simulink model "car_model_5_28_2023"  (R2022b)
settings: Solver=VariableStepAuto  StartTime=0.0  StopTime=15  RelTol=1e-3
values from neighbouring files (symbols this model uses):
  dZ = 0.295    [Startup.m]
  F0z = [0 0]    [Startup.m]
  phi = 45    [Startup.m]
  X = Reference_Signals.Chassis_Position.X.Data(:)    [Simulation_Data_Parse.m]    (also in Vehicle_Sim_Parse.m = Chassis_Signals.InertFrm.Cg.Disp.X.Data(:))
  Y = Reference_Signals.Chassis_Position.Y.Data(:)    [Simulation_Data_Parse.m]    (also in Vehicle_Sim_Parse.m = Chassis_Signals.InertFrm.Cg.Disp.Y.Data(:))
undefined symbols (not defined in the file or in its folder): chassis, DiscIntNeverNeededParam, driver, IMU_accel, IMU_gyro, IMU_mag, powertrain, psi, sensor, sim, sus, suspension, theta, trn, tvs, veh, VEH, whl, Xdot, Ydot, Z, Zdot
libraries: fl_lib x53, nesl_utility x15, vehdynlibtire x10, vehdynlibsuspension x8, EngineCoolingComponents_lib x5, autolibutils x5, sharedtransform x5, dspstat3 x2, simulink x2, slpidlib x2, shared6dof x2, sensorgpslib x1
(part 2 of 9)

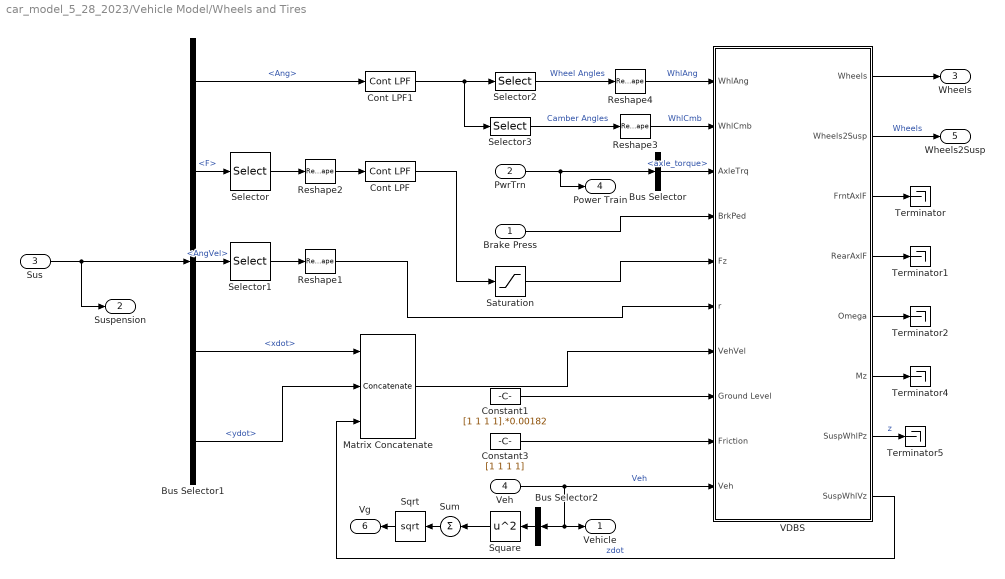
== system car_model_5_28_2023/Vehicle Model/Wheels and Tires ==
  Brake Press : Inport  Unit=Pa
  PwrTrn : Inport  Port=2
  Sus : Inport  Port=3
  Veh : Inport  Port=4
  Bus Selector : BusSelector  OutputSignals=axle_torque
  Bus Selector1 : BusSelector  OutputSignals=Whl.Ang,Whl.F,Whl.AngVel,Whl.xdot,Whl.ydot
  Bus Selector2 : BusSelector  OutputSignals=BdyFrm.Cg.Vel.xdot,BdyFrm.Cg.Vel.ydot  OutputAsBus=on
  Constant1 : Constant  Value=[1 1 1 1].*0.00182
  Constant3 : Constant  Value=[1 1 1 1]
  Cont LPF : autolibutils/Cont LPF  wc=100*2*pi  AbsoluteTolerance=auto  aMode=2
  Cont LPF1 : autolibutils/Cont LPF  wc=100*2*pi  AbsoluteTolerance=auto  aMode=2
  Matrix Concatenate : Concatenate  NumInputs=3  Mode=Multidimensional array
  Reshape{1..4} (4 alike) : Reshape
  Saturation : Saturate  UpperLimit=inf  LowerLimit=-10*9.81*2000  ZeroCross=off
  Selector : Selector  NumberOfDimensions=2  InputPortWidth=3  IndexOptions=Index vector (dialog),Select all  Indices=[3],1  OutputSizes=1,1
  Selector1 : Selector  NumberOfDimensions=2  InputPortWidth=1  IndexOptions=Index vector (dialog),Select all  Indices=[3],1  OutputSizes=1,1
  Selector2 : Selector  NumberOfDimensions=2  InputPortWidth=3  IndexOptions=Index vector (dialog),Select all  Indices=3,1  OutputSizes=1,1
  Selector3 : Selector  NumberOfDimensions=2  InputPortWidth=3  IndexOptions=Index vector (dialog),Select all  Indices=1,1  OutputSizes=1,1
  Sqrt : Sqrt
  Square : Math  Operator=square
  Sum : Sum  Inputs=+
  Terminator{,1..2,4..5} (5 alike) : Terminator
  VDBS : Subsystem  VariantControl=0
  Vehicle : Outport  VectorParamsAs1DForOutWhenUnconnected=off
  Suspension : Outport  Port=2  VectorParamsAs1DForOutWhenUnconnected=off
  Wheels : Outport  Port=3  VectorParamsAs1DForOutWhenUnconnected=off
  Power Train : Outport  Port=4  VectorParamsAs1DForOutWhenUnconnected=off
  Wheels2Susp : Outport  Port=5  VectorParamsAs1DForOutWhenUnconnected=off
  Vg : Outport  Port=6  VectorParamsAs1DForOutWhenUnconnected=off
  wires:
  Bus Selector1/2 -> Selector/1  "<F>"
  VDBS/3(FrntAxlF) -> Terminator/1
  VDBS/4(RearAxlF) -> Terminator1/1
  VDBS/6(Mz) -> Terminator4/1
  Selector1/1 -> Reshape1/1
  Matrix Concatenate/1 -> VDBS/7(VehVel)
  PwrTrn/1 -> Power Train/1, Bus Selector/1
  Reshape4/1 -> VDBS/1(WhlAng)  "WhlAng"
  Reshape3/1 -> VDBS/2(WhlCmb)  "WhlCmb"
  Selector/1 -> Reshape2/1
  Saturation/1 -> VDBS/5(Fz)
  Constant1/1 -> VDBS/8(Ground Level)
  VDBS/8(SuspWhlVz) -> Matrix Concatenate/3  "zdot"
  Bus Selector1/1 -> Cont LPF1/1  "<Ang>"
  Selector3/1 -> Reshape3/1  "Camber Angles"
  Sus/1 -> Suspension/1, Bus Selector1/1
  Bus Selector1/4 -> Matrix Concatenate/1  "<xdot>"
  Bus Selector1/5 -> Matrix Concatenate/2  "<ydot>"
  VDBS/7(SuspWhlPz) -> Terminator5/1  "z"
  Reshape2/1 -> Cont LPF/1
  Bus Selector1/3 -> Selector1/1  "<AngVel>"
  Reshape1/1 -> VDBS/6(r)
  Brake Press/1 -> VDBS/4(BrkPed)
  Constant3/1 -> VDBS/9(Friction)
  Cont LPF/1 -> Saturation/1
  Cont LPF1/1 -> Selector3/1, Selector2/1
  Selector2/1 -> Reshape4/1  "Wheel Angles"
  Veh/1 -> Vehicle/1, Bus Selector2/1, VDBS/10(Veh)  "Veh"
  VDBS/2(Wheels2Susp) -> Wheels2Susp/1  "Wheels"
  VDBS/1(Wheels) -> Wheels/1
  Bus Selector/1 -> VDBS/3(AxleTrq)  "<axle_torque>"
  VDBS/5(Omega) -> Terminator2/1
  Bus Selector2/1 -> Square/1
  Square/1 -> Sum/1
  Sum/1 -> Sqrt/1
  Sqrt/1 -> Vg/1

== system car_model_5_28_2023/Control Systems/TVS/Current Limiting ==
  omega : Inport
  k_TV : Inport  Port=2
  2-D Lookup Table : Lookup_n-D  LookupTableObject=''  BreakpointsForDimension1=tvs.torque_control.omega_bp  BreakpointsForDimension2=tvs.torque_control.k_linear_bp  BreakpointsForDimension1FirstPoint=10  BreakpointsForDimension2FirstPoint=10  BreakpointsForDimension1Spacing=12  BreakpointsForDimension2Spacing=12  Table=tvs.torque_control.k_actual  ExtrapMethod=Clip  DiagnosticForOutOfRangeInput=Error  InternalRulePriority=Speed  RndMeth=Simplest
      settings: InputPortMap=u0,u1
  Gain1 : Gain  Gain=powertrain.gearbox.gr
  K_Actual : Outport
  wires:
  2-D Lookup Table/1 -> K_Actual/1
  k_TV/1 -> 2-D Lookup Table/2
  omega/1 -> Gain1/1
  Gain1/1 -> 2-D Lookup Table/1

== system car_model_5_28_2023/Control Systems/TVS/Optimization ==
  note: reduce this limit?
  driver_input : Inport  OutDataTypeStr=double
  obj_gain : Inport  Port=2
  b : Inport  Port=3  OutDataTypeStr=double
  ub : Inport  Port=4  OutDataTypeStr=double
  lb : Inport  Port=5  OutDataTypeStr=double
  Aeq : Inport  Port=6  OutDataTypeStr=double
  beq : Inport  Port=7  OutDataTypeStr=double
  A Dot : DotProduct  OutDataTypeStr=double
  Aeq Dot : DotProduct  OutDataTypeStr=double
  C Caller : CCaller  FunctionName=bigM_func
  Constant : Constant  Value=sim.top_parameters.TVS_ENABLE
  Constant1 : Constant  Value=[1 1 1 1]
  Demux{,1..4} (5 alike) : Demux
  Switch : Switch  Criteria=u2 > Threshold  SaturateOnIntegerOverflow=off  InputSameDT=off
  Tx_RAW_demux : Mux
  Tx_choose : Switch  Criteria=u2 > Threshold  Threshold=2  OutDataTypeStr=double  SaturateOnIntegerOverflow=off  InputSameDT=off
  Tx_deadband : DeadZone  LowerValue=-10*tvs.power_control.dTx  UpperValue=10*tvs.power_control.dTx
  Tx_equal_gain : Gain  Gain=tvs.power_control.ABS_MAX_TORQUE.*sim.top_parameters.MOTOR_ENABLE  OutDataTypeStr=double
  Tx_equal_offset : Bias  Bias=tvs.power_control.ABS_MAX_TORQUE  SaturateOnIntegerOverflow=off
  Tx_initial : Constant  Value=0  OutDataTypeStr=double
  Tx_reverse_offset : Bias  Bias=-tvs.power_control.ABS_MAX_TORQUE  SaturateOnIntegerOverflow=off
  b Add : Sum  OutDataTypeStr=double
  beq Add : Sum  OutDataTypeStr=double
  lb_offset : Bias  Bias=tvs.power_control.ABS_MAX_TORQUE  SaturateOnIntegerOverflow=off
  optimization_offset_A : Constant  Value=tvs.power_control.ABS_MAX_TORQUE  OutDataTypeStr=double
  optimization_offset_Aeq : Constant  Value=tvs.power_control.ABS_MAX_TORQUE  OutDataTypeStr=double
  ub_offset : Bias  Bias=tvs.power_control.ABS_MAX_TORQUE  SaturateOnIntegerOverflow=off
  yaw_error_limit : Constant  Value=tvs.yaw_control.dy  OutDataTypeStr=double
  Tx : Outport
  exitflag : Outport  Port=2
  wires:
  C Caller/1 -> Tx_choose/2, exitflag/1  "exitflag"
  lb/1 -> lb_offset/1  "lb"
  ub/1 -> ub_offset/1  "ub"
  C Caller/2 -> Tx_RAW_demux/1  "TFL"
  C Caller/5 -> Tx_RAW_demux/4  "TRR"
  C Caller/4 -> Tx_RAW_demux/3  "TRL"
  C Caller/3 -> Tx_RAW_demux/2  "TFR"
  Demux/1 -> C Caller/1  "obj_FL"
  Demux/2 -> C Caller/2  "obj_FR"
  Demux/3 -> C Caller/3  "obj_RL"
  Demux/4 -> C Caller/4  "obj_RR"
  Tx_initial/1 -> C Caller/23, C Caller/24, C Caller/25, C Caller/26  "Tx_initial"
  Demux1/1 -> C Caller/19  "ub_FL"
  Demux1/2 -> C Caller/20  "ub_FR"
  Demux1/3 -> C Caller/21  "ub_RL"
  Demux1/4 -> C Caller/22  "ub_RR"
  Demux2/1 -> C Caller/15  "lb_FL"
  Demux2/2 -> C Caller/16  "lb_FR"
  Demux2/3 -> C Caller/17  "lb_RL"
  Demux2/4 -> C Caller/18  "lb_RR"
  Demux3/3 -> C Caller/13  "Aeq_RL"
  Demux3/2 -> C Caller/12  "Aeq_FR"
  Demux3/1 -> C Caller/11  "Aeq_FL"
  Demux3/4 -> C Caller/14  "Aeq_RR"
  Demux4/1 -> C Caller/6  "A_FL"
  Demux4/2 -> C Caller/7  "A_FR"
  Demux4/3 -> C Caller/8  "A_RL"
  Demux4/4 -> C Caller/9  "A_RR"
  ub_offset/1 -> Demux1/1  "ub_b"
  optimization_offset_Aeq/1 -> Aeq Dot/1  "offset"
  optimization_offset_A/1 -> A Dot/1  "offset"
  beq/1 -> beq Add/1  "beq"
  Aeq Dot/1 -> beq Add/2  "Aeq_b"
  b/1 -> b Add/1  "b"
  A Dot/1 -> b Add/2
  yaw_error_limit/1 -> C Caller/27  "yaw_error_limit"
  Tx_RAW_demux/1 -> Tx_choose/1  "Tx_RAW_TV"
  Constant1/1 -> Demux4/1, A Dot/2  "A"
  b Add/1 -> C Caller/5  "b_b"
  obj_gain/1 -> Demux/1  "obj_gain"
  lb_offset/1 -> Demux2/1  "lb_b"
  Aeq/1 -> Demux3/1, Aeq Dot/2  "Aeq"
  beq Add/1 -> C Caller/10  "beq_b"
  Tx_deadband/1 -> Tx/1  "Tx"
  Tx_reverse_offset/1 -> Tx_deadband/1
  driver_input/1 -> Tx_equal_gain/1
  Tx_choose/1 -> Switch/1
  Tx_equal_gain/1 -> Tx_equal_offset/1  "Tx_equal"
  Tx_equal_offset/1 -> Switch/3, Tx_choose/3
  Switch/1 -> Tx_reverse_offset/1
  Constant/1 -> Switch/2

== system car_model_5_28_2023/Control Systems/TVS/Power Controller ==
  note: Max Throttle as Limit or Max Current as limit?
  note: Tune the endpoints
  vel : Inport  OutDataTypeStr=double
  battery_voltage : Inport  Port=2
  dcl : Inport  Port=3  OutDataTypeStr=double  LockScale=on
  ccl : Inport  Port=4  OutDataTypeStr=double  LockScale=on
  driver_input : Inport  Port=5  OutDataTypeStr=double  LockScale=on
  motor_temp : Inport  Port=6
  mc_temp : Inport  Port=7
  omega : Inport  Port=8
  In9 : Inport  Port=9
  Constant2 : Constant  Value=tvs.power_control.ABS_MIN_TORQUE  OutDataTypeStr=double
  Constant3 : Constant  Value=tvs.power_control.ABS_MAX_TORQUE
  Current to RAW Throttle : Gain  Gain=tvs.power_control.ABS_MAX_TRQ_CMD/tvs.power_control.ABS_MAX_I_FLOW
  Gain : Gain  Gain=tvs.power_control.ABS_MAX_I_FLOW
  Gain4 : Gain  Gain=-sim.top_parameters.MOTOR_ENABLE  ParamDataTypeStr=double  OutDataTypeStr=Inherit: Inherit via back propagation
  Gain8 : Gain  Gain=sim.top_parameters.MOTOR_ENABLE  ParamDataTypeStr=double  OutDataTypeStr=Inherit: Inherit via back propagation
  Max : MinMax  Function=max
  Max Torque : Saturate  UpperLimit=tvs.power_control.ABS_MAX_TORQUE  LowerLimit=2.*tvs.power_control.dTx  OutDataTypeStr=Inherit: Inherit via back propagation
  Max1 : MinMax  Function=max
  Min Torque : Saturate  UpperLimit=tvs.power_control.dTx  LowerLimit=tvs.power_control.ABS_MIN_TORQUE  OutDataTypeStr=Inherit: Inherit via back propagation
  Minimum : MinMax  Inputs=4
  Saturation1 : Saturate  UpperLimit=tvs.power_control.ABS_MAX_TRQ_CMD  LowerLimit=tvs.power_control.ABS_MIN_TRQ_CMD
  Selector : Selector  InputPortWidth=4  IndexOptions=Index vector (dialog)  Indices=4  OutputSizes=1
  Switch1 : Switch  Threshold=tvs.power_control.min_velocity_regen  OutDataTypeStr=Inherit: Inherit via back propagation  SaturateOnIntegerOverflow=off  InputSameDT=off
  Temperature to Motor Controller Current Limit Map : Lookup_n-D  NumberOfTableDimensions=1  BreakpointsForDimension1=tvs.power_control.motor_controller_t_bp  IndexSearchMethod=Evenly spaced points  Table=tvs.power_control.motor_controller_I_table  ExtrapMethod=Clip  UseLastTableValue=on  InternalRulePriority=Speed  RndMeth=Simplest
  Temperature to Motor Current Limit Map : Lookup_n-D  NumberOfTableDimensions=1  BreakpointsForDimension1=tvs.power_control.motor_t_bp  IndexSearchMethod=Evenly spaced points  Table=tvs.power_control.motor_I_table  ExtrapMethod=Clip  UseLastTableValue=on  InternalRulePriority=Speed  RndMeth=Simplest
  Terminator : Terminator
  Terminator1 : Terminator
  Terminator2 : Terminator
  b : Outport  OutDataTypeStr=double  LockScale=on
  ub : Outport  Port=2  OutDataTypeStr=double  LockScale=on
  lb : Outport  Port=3  OutDataTypeStr=double  LockScale=on
  wires:
  Max1/1 -> Temperature to Motor Controller Current Limit Map/1
  Temperature to Motor Current Limit Map/1 -> Minimum/2  "Total Motor Current Limit (A)"
  battery_voltage/1 -> Terminator1/1
  Gain8/1 -> Max Torque/1
  Constant3/1 -> Gain4/1, Gain8/1
  Max/1 -> Temperature to Motor Current Limit Map/1
  Gain4/1 -> Min Torque/1
  Constant2/1 -> Switch1/3  "Abs Min Torque CMD"
  Selector/1 -> Switch1/2  "Planer Vcog (m/s)"
  motor_temp/1 -> Max/1  "[FL FR RL RR] Motor Temperature (degC)"
  ccl/1 -> Terminator/1
  driver_input/1 -> Gain/1  "RAW Throttle"
  Max Torque/1 -> ub/1  "Max Individual Motor Torque (Nm)"
  Gain/1 -> Minimum/1
  mc_temp/1 -> Max1/1  "[FL FR RL RR] Motor Controller Temperature (degC)"
  dcl/1 -> Minimum/4  "Discharge Current Limit (A)"
  vel/1 -> Selector/1  "[Vx Vy Vcog]"
  Temperature to Motor Controller Current Limit Map/1 -> Minimum/3  "Total Motor Controller Current Limit (A)"
  Min Torque/1 -> Switch1/1
  Switch1/1 -> lb/1  "Min Individual Motor Torque (Nm)"
  Minimum/1 -> Current to RAW Throttle/1  "Max Allowed Current (A)"
  omega/1 -> Terminator2/1
  Saturation1/1 -> b/1  "Limited Total Torque Request (Nm)"
  Current to RAW Throttle/1 -> Saturation1/1  "Torque CMD (Nm)"

== system car_model_5_28_2023/Control Systems/TVS/Traction Controller ==
  Fz : Inport  OutDataTypeStr=double  LockScale=on
  vel : Inport  Port=2  OutDataTypeStr=double  LockScale=on
  ang_vel : Inport  Port=3  OutDataTypeStr=double  LockScale=on
  CCSA : Inport  Port=4
  omega : Inport  Port=5
  1-D Lookup Table : Lookup_n-D  NumberOfTableDimensions=1  BreakpointsForDimension1=suspension.tire.Fz_sweep  Table=suspension.tire.cy_sweep  InternalRulePriority=Speed  RndMeth=Simplest
  1-D Lookup Table1 : Lookup_n-D  NumberOfTableDimensions=1  BreakpointsForDimension1=suspension.tire.Fz_sweep  Table=suspension.tire.my_sweep  InternalRulePriority=Speed  RndMeth=Simplest
  1-D Lookup Table2 : Lookup_n-D  NumberOfTableDimensions=1  BreakpointsForDimension1=suspension.tire.Fz_sweep  Table=suspension.tire.kx_sweep  InternalRulePriority=Speed  RndMeth=Simplest
  1-D Lookup Table3 : Lookup_n-D  NumberOfTableDimensions=1  BreakpointsForDimension1=suspension.tire.Fz_sweep  Table=suspension.tire.mx_sweep  InternalRulePriority=Speed  RndMeth=Simplest
  Compute SA : Subsystem
  Compute SL : Subsystem
  Compute SL Fake : Subsystem
  Constant : Constant
  Constant1 : Constant  Value=[1 1 1 1].*tvs.traction_control.low_V_SA
  Constant2 : Constant  Value=sim.top_parameters.TRACTION_ENABLE
  Divide : Product  Inputs=**//
  Divide1 : Product  Inputs=**//
  Gain : Gain  Gain=powertrain.gearbox.gr./suspension.tire.RE
  Selector : Selector  InputPortWidth=4  IndexOptions=Index vector (dialog)  Indices=4  OutputSizes=1
  Selector1 : Selector  InputPortWidth=4  IndexOptions=Index vector (dialog)  Indices=4  OutputSizes=1
  Sqrt : Sqrt
  Square : Math  Operator=square
  Square1 : Math  Operator=square
  Steering Model : Subsystem
  Sum : Sum  Inputs=|++
  Switch : Switch  Criteria=u2 > Threshold  Threshold=tvs.traction_control.Vth  SaturateOnIntegerOverflow=off  InputSameDT=off
  Switch1 : Switch  Criteria=u2 > Threshold  Threshold=tvs.traction_control.Vth  SaturateOnIntegerOverflow=off  InputSameDT=off
  Switch2 : Switch  Criteria=u2 > Threshold  SaturateOnIntegerOverflow=off  InputSameDT=off
  obj_gain : Outport
  wires:
  Gain/1 -> obj_gain/1  "obj_gain"
  Constant/1 -> Gain/1, Switch2/3
  Sum/1 -> Sqrt/1
  Divide/1 -> Square/1  "a_bar"
  1-D Lookup Table/1 -> Divide/2
  1-D Lookup Table1/1 -> Divide/3
  Fz/1 -> 1-D Lookup Table1/1, Divide/4, 1-D Lookup Table2/1, 1-D Lookup Table3/1, Divide1/4, 1-D Lookup Table/1
  Divide1/1 -> Square1/1  "s_bar"
  1-D Lookup Table2/1 -> Divide1/2
  1-D Lookup Table3/1 -> Divide1/3
  Switch/1 -> Divide1/1
  Switch1/1 -> Divide/1
  Compute SL Fake/1(SL_fake) -> Switch/3
  Compute SL/1(Out1) -> Switch/1
  Compute SA/1(Out1) -> Switch1/1, Compute SL/1(In1)
  vel/1 -> Compute SL/3(Vg), Selector/1, Compute SL Fake/2(Vg), Selector1/1, Compute SA/3(Vg)
  ang_vel/1 -> Compute SA/2(ang_vel)
  omega/1 -> Compute SL Fake/1(omega), Compute SL/2(omega)
  Steering Model/1(steering) -> Compute SA/1(steering)
  Constant1/1 -> Switch1/3
  Sqrt/1 -> Switch2/1
  Constant2/1 -> Switch2/2
  Selector/1 -> Switch/2
  Selector1/1 -> Switch1/2
  Square/1 -> Sum/1
  Square1/1 -> Sum/2
  CCSA/1 -> Steering Model/1(steering_angle)

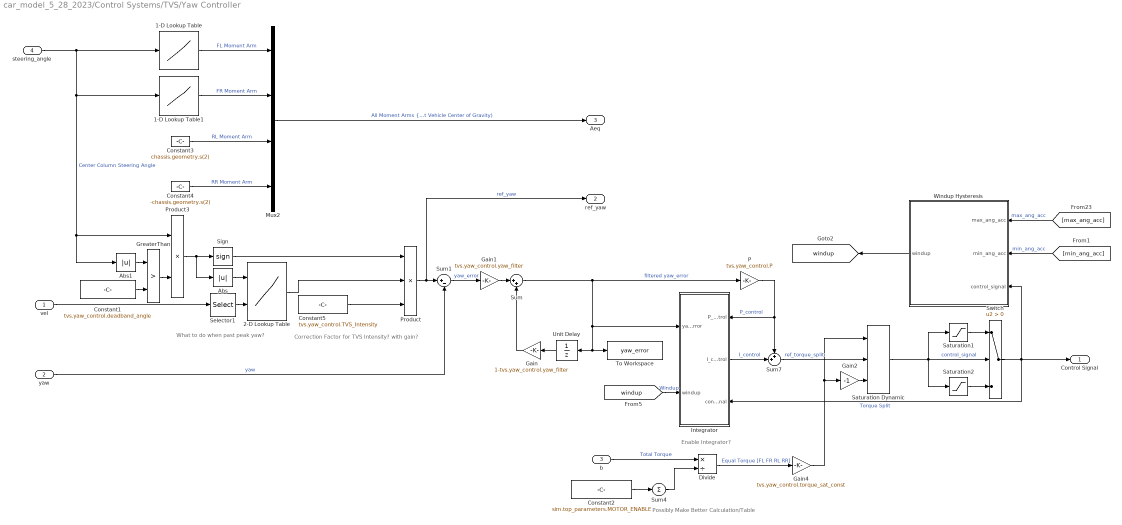
== system car_model_5_28_2023/Control Systems/TVS/Yaw Controller ==
  note: Correction Factor for TVS Intensity? with gain?
  note: Enable Integrator?
  note: What to do when past peak yaw?
  note: Possibly Make Better Calculation/Table
  vel : Inport
  yaw : Inport  Port=2  OutDataTypeStr=double  LockScale=on
  b : Inport  Port=3
  steering_angle : Inport  Port=4
  1-D Lookup Table : Lookup_n-D  NumberOfTableDimensions=1  BreakpointsForDimension1=suspension.steering.theta_sweep  Table=suspension.steering.Aeq_left  ExtrapMethod=Clip  InternalRulePriority=Speed  RndMeth=Simplest
  1-D Lookup Table1 : Lookup_n-D  NumberOfTableDimensions=1  BreakpointsForDimension1=suspension.steering.theta_sweep  Table=suspension.steering.Aeq_right  ExtrapMethod=Clip  InternalRulePriority=Speed  RndMeth=Simplest
  2-D Lookup Table : Lookup_n-D  BreakpointsForDimension1=tvs.yaw_control.max_s_bp  BreakpointsForDimension2=tvs.yaw_control.max_v_bp  Table=tvs.yaw_control.max_yaw_table_ref  ExtrapMethod=Clip  InternalRulePriority=Speed  RndMeth=Simplest
      settings: InputPortMap=u0,u1
  Abs : Abs  SaturateOnIntegerOverflow=off
  Abs1 : Abs  SaturateOnIntegerOverflow=off
  Constant1 : Constant  Value=tvs.yaw_control.deadband_angle
  Constant2 : Constant  Value=sim.top_parameters.MOTOR_ENABLE
  Constant3 : Constant  Value=chassis.geometry.s(2)  OutDataTypeStr=Inherit: Inherit via back propagation
  Constant4 : Constant  Value=-chassis.geometry.s(2)  OutDataTypeStr=Inherit: Inherit via back propagation
  Constant5 : Constant  Value=tvs.yaw_control.TVS_Intensity
  Divide : Product  Inputs=*/
  Gain : Gain  Gain=1-tvs.yaw_control.yaw_filter
  Gain1 : Gain  Gain=tvs.yaw_control.yaw_filter
  Gain2 : Gain  Gain=-1
  Gain4 : Gain  Gain=tvs.yaw_control.torque_sat_const
  GreaterThan : RelationalOperator  Operator=>  OutDataTypeStr=boolean  RndMeth=Simplest  InputSameDT=off
  Integrator : Subsystem
      settings: PortSchema="{\"entries\":[{\"content\":{\"sides\":[{\"content\":{\"connectorIds\":[\"In1\",\"In2\"]},\"type\":\"ConnectorPlacement.EquallySpacedRectSide\",\"uuid\":\"8eceed30-5463-482b-9ad9-1d0859eec1e0\"},{\"content\":{\"connectorIds\":[\"In3\",\"Out1\",\"In4\"],\"side\":\"RIGHT\"},\"type\":\"ConnectorPlacement.EquallySpacedRectSide\",\"uuid\":\"ca18b8b2-b2b4-4da4-8362-ca68ae703b33\"},{\"content\":{\"connectorIds\":[],\"side\":\"TOP\"},\"type\":\"ConnectorPlacement.EquallySpacedRectSide\",\"uuid\":\"14e81d29-e47e-408e-961b-b14eadc3d40e\"}]},\"type\":\"ConnectorPlacement.EquallySpacedConnector\",\"uuid\":\"147d3fcd-d0df-4d8b-910b-d1c7e2c77e1f\"}],\"packageUris\":[\"http://schema.mathworks.com/mf0/Connector/R2020b\"],\"version\":\"1.0\"}"
  Mux2 : Mux
  P : Gain  Gain=tvs.yaw_control.P  ParamDataTypeStr=double  OutDataTypeStr=double
  Product : Product  Inputs=3  OutDataTypeStr=Inherit: Inherit via back propagation
  Product3 : Product
  Saturation Dynamic : simulink/Discontinuities/Saturation Dynamic  OutMin=[]  OutMax=[]  OutDataTypeStr=Inherit: Same as second input  OutDataType=fixdt(1, 16)  OutScaling=2^-10  DoSatur=off
  Saturation1 : Saturate  UpperLimit=inf  LowerLimit=tvs.yaw_control.dB
  Saturation2 : Saturate  UpperLimit=-tvs.yaw_control.dB  LowerLimit=-inf
  Selector1 : Selector  InputPortWidth=4  IndexOptions=Index vector (dialog)  Indices=4  OutputSizes=1
  Sign : Signum
  Sum : Sum  Inputs=|++
  Sum1 : Sum  Inputs=|+-  OutDataTypeStr=Inherit: Inherit via back propagation
  Sum4 : Sum  Inputs=+
  Sum7 : Sum  Inputs=++|  OutDataTypeStr=double  SaturateOnIntegerOverflow=on
  Switch : Switch  Criteria=u2 > Threshold  SaturateOnIntegerOverflow=off  InputSameDT=off
  To Workspace : ToWorkspace  VariableName=yaw_error  SaveFormat=Timeseries  SampleTime=-1
  Unit Delay : UnitDelay  SampleTime=-1  HasFrameUpgradeWarning=on
  Windup Hysteresis : Subsystem
  Control Signal : Outport  OutDataTypeStr=double  PortDimensions=1  LockScale=on
  ref_yaw : Outport  Port=2
  Aeq : Outport  Port=3  OutDataTypeStr=double  LockScale=on
  tag scope: windup=global
  wires:
  P/1 -> Sum7/1, Integrator/3(P_control)  "P_control"
  yaw/1 -> Sum1/2  "yaw"
  Integrator/1(I_control) -> Sum7/2  "I_control"
  Sum7/1 -> Saturation Dynamic/2  "ref_torque_split"
  Saturation Dynamic/1 -> Saturation2/1, Saturation1/1, Switch/2  "control_signal"
  Windup Hysteresis/1(windup) -> [windup]
  Sum/1 -> P/1, Unit Delay/1, To Workspace/1, Integrator/1(yaw_error)  "filtered yaw_error"
  [windup] -> Integrator/2(windup)  "Windup"
  Unit Delay/1 -> Gain/1
  Gain/1 -> Sum/2
  Gain1/1 -> Sum/1
  Sum1/1 -> Gain1/1  "yaw_error"
  Switch/1 -> Windup Hysteresis/3(control_signal), Control Signal/1, Integrator/4(control_signal)  "Torque Split"
  Saturation1/1 -> Switch/1
  Saturation2/1 -> Switch/3
  Constant4/1 -> Mux2/4  "RR Moment Arm"
  b/1 -> Divide/1  "Total Torque"
  Constant3/1 -> Mux2/3  "RL Moment Arm"
  1-D Lookup Table/1 -> Mux2/1  "FL Moment Arm"
  1-D Lookup Table1/1 -> Mux2/2  "FR Moment Arm"
  Mux2/1 -> Aeq/1  "All Moment Arms {FL FR RL RR] (about Vehicle Center of Gravity)"
  Divide/1 -> Gain4/1  "Equal Torque [FL FR RL RR]"
  Product/1 -> ref_yaw/1, Sum1/1  "ref_yaw"
  Constant1/1 -> GreaterThan/2
  steering_angle/1 -> 1-D Lookup Table1/1, Product3/1, Abs1/1, 1-D Lookup Table/1  "Center Column Steering Angle"
  vel/1 -> Selector1/1
  Abs/1 -> 2-D Lookup Table/1
  Product3/1 -> Abs/1, Sign/1
  Sign/1 -> Product/1
  Abs1/1 -> GreaterThan/1
  GreaterThan/1 -> Product3/2
  Selector1/1 -> 2-D Lookup Table/2
  [min_ang_acc] -> Windup Hysteresis/2(min_ang_acc)  "min_ang_acc"
  [max_ang_acc] -> Windup Hysteresis/1(max_ang_acc)  "max_ang_acc"
  Gain2/1 -> Saturation Dynamic/3
  Gain4/1 -> Gain2/1, Saturation Dynamic/1
  2-D Lookup Table/1 -> Product/2
  Constant5/1 -> Product/3
  Constant2/1 -> Sum4/1
  Sum4/1 -> Divide/2

== system car_model_5_28_2023/Driver & Environment/Lateral Control/Steady State Model ==
  <yaw_ref> : Inport
  <v_cog> : Inport  Port=2
  1-D Lookup Table : Lookup_n-D  NumberOfTableDimensions=1  BreakpointsForDimension1=driver.control.max_v_bp  Table=driver.control.max_yaw_table  ExtrapMethod=Clip  InternalRulePriority=Speed  RndMeth=Simplest
  1-D Lookup Table1 : Lookup_n-D  NumberOfTableDimensions=1  BreakpointsForDimension1=driver.control.max_v_bp  Table=driver.control.max_theta_table  InternalRulePriority=Speed  RndMeth=Simplest
  2-D Lookup Table1 : Lookup_n-D  BreakpointsForDimension1=driver.control.max_y_bp  BreakpointsForDimension2=driver.control.max_v_bp  Table=driver.control.steering_angle_table  ExtrapMethod=Clip  InternalRulePriority=Speed  RndMeth=Simplest
      settings: InputPortMap=u0,u1
  Abs : Abs  SaturateOnIntegerOverflow=off
  Min : MinMax  Inputs=2
  Min1 : MinMax  Inputs=2
  Product : Product
  Sign : Signum
  Sign Angle : Outport
  steady State Angle : Outport  Port=2
  wires:
  Sign/1 -> Sign Angle/1, Product/1
  1-D Lookup Table1/1 -> Min/2
  Min1/1 -> 2-D Lookup Table1/1
  <yaw_ref>/1 -> Abs/1, Sign/1
  <v_cog>/1 -> 2-D Lookup Table1/2, 1-D Lookup Table1/1, 1-D Lookup Table/1
  Min/1 -> Product/2
  Abs/1 -> Min1/2
  2-D Lookup Table1/1 -> Min/1
  Product/1 -> steady State Angle/1
  1-D Lookup Table/1 -> Min1/1

== system car_model_5_28_2023/Driver & Environment/Longitudinal Control/AAS ==
  note: simple proportional controller for speed control
  omega : Inport
  v_error : Inport  Port=2
  Dead Zone : DeadZone  LowerValue=-15  UpperValue=15
  Discrete Derivative : simulink/Discrete/Discrete Derivative  gainval=1.0  ICPrevScaledInput=0.0  OutMin=[]  OutMax=[]  OutDataType=fixdt(1, 16)  OutScaling=2^-10  DoSatur=off
  Discrete-Time Integrator : DiscreteIntegrator  ExternalReset=either  SampleTime=-1  ICPrevOutput=DiscIntNeverNeededParam  ICPrevScaledInput=DiscIntNeverNeededParam
  Gain : Gain  Gain=driver.control.P_Driver
  Gain1 : Gain  Gain=1/20
  Max : MinMax  Function=max
  Saturation : Saturate  UpperLimit=sim.range.Max_Driver_Input  LowerLimit=sim.range.Min_Driver_Input
  Saturation1 : Saturate  UpperLimit=inf  LowerLimit=0
  Sign : Signum
  Terminator : Terminator
  driver_input : Outport
  wires:
  Gain/1 -> Saturation/1
  v_error/1 -> Gain/1  "v_error"
  omega/1 -> Discrete Derivative/1
  Discrete Derivative/1 -> Dead Zone/1
  Discrete-Time Integrator/1 -> Max/1
  Dead Zone/1 -> Sign/1, Discrete-Time Integrator/1
  Sign/1 -> Discrete-Time Integrator/2
  Max/1 -> Saturation1/1
  Saturation1/1 -> Gain1/1
  Gain1/1 -> Terminator/1
  Saturation/1 -> driver_input/1

== system car_model_5_28_2023/Driver & Environment/Longitudinal Control/ABS ==
  yaw : Inport
  Fz : Inport  Port=2
  ABS_ENABLE : Inport  Port=3
  1-D Lookup Table : Lookup_n-D  NumberOfTableDimensions=1  BreakpointsForDimension1=[0;200;400;600;800;1000;1200]  Table=[0;0;500000;750000;1000000;2000000;2000000]  ExtrapMethod=Clip  InternalRulePriority=Speed  RndMeth=Simplest
  Dead Zone : DeadZone  LowerValue=-0.1  UpperValue=0.1
  Gain : Gain  Gain=0.25
  Gain3 : Gain  Gain=1-driver.control.pressure_filter
  Gain4 : Gain  Gain=driver.control.pressure_filter*sim.top_parameters.YAW_ENABLE*driver.control.brake_gain
  Left Turn : Mux
  Min : MinMax  Inputs=2
  Min1 : MinMax
  Min2 : MinMax
  NOT : Logic  Operator=NOT  IconShape=distinctive  AllPortsSameDT=off  OutDataTypeStr=boolean
  Product1 : Product
  Right Turn : Mux
  Saturation2 : Saturate  UpperLimit=sim.range.Max_Brake_Pressure  LowerLimit=sim.range.Min_Brake_Pressure
  Selector2 : Selector  InputPortWidth=4  IndexOptions=Index vector (dialog)  Indices=[1 2]  OutputSizes=1
  Straight : Mux
  Sum2 : Sum  Inputs=|++
  Switch : Switch  Criteria=u2 ~= 0  SaturateOnIntegerOverflow=off  InputSameDT=off
  Switch1 : Switch  Criteria=u2 > Threshold  SaturateOnIntegerOverflow=off  InputSameDT=off
  Unit Delay1 : UnitDelay  SampleTime=-1  HasFrameUpgradeWarning=on
  Px : Outport
  wires:
  ABS_ENABLE/1 -> Product1/1
  Gain3/1 -> Sum2/2
  Unit Delay1/1 -> Gain3/1
  Gain4/1 -> Sum2/1
  Sum2/1 -> Saturation2/1, Unit Delay1/1
  Fz/1 -> Product1/2
  Saturation2/1 -> Px/1
  Product1/1 -> 1-D Lookup Table/1
  Gain/1 -> Min/1
  1-D Lookup Table/1 -> Min2/1, Selector2/1
  Selector2/1 -> Min1/1
  Min1/1 -> Straight/2, Right Turn/3, Left Turn/2, Left Turn/4, Right Turn/1, Straight/1, Gain/1
  Min/1 -> Left Turn/1, Left Turn/3, Right Turn/4, Right Turn/2, Straight/4, Straight/3
  Min2/1 -> Min/2
  Straight/1 -> Switch/1
  Left Turn/1 -> Switch1/3
  Right Turn/1 -> Switch1/1
  Switch1/1 -> Switch/3
  Switch/1 -> Gain4/1
  yaw/1 -> Dead Zone/1
  Dead Zone/1 -> Switch1/2, NOT/1
  NOT/1 -> Switch/2

== system car_model_5_28_2023/Driver & Environment/Longitudinal Control/Pedal Positioner ==
  note: Determine when it is ok to trigger braking. If velocity error less than 0 (want to brake) and driver input is 0 (ready to brake) and not turning then it is ok to trigger brake
  <v_error> : Inport
  driver_input : Inport  Port=2
  AND : Logic  IconShape=distinctive  AllPortsSameDT=off  OutDataTypeStr=boolean
  Constant6 : Constant  Value=0
  Less Than1 : RelationalOperator  Operator=<=  OutDataTypeStr=boolean  RndMeth=Simplest  InputSameDT=off
  Less Than2 : RelationalOperator  Operator=<  OutDataTypeStr=boolean  RndMeth=Simplest  InputSameDT=off
  brake : Outport
  wires:
  Constant6/1 -> Less Than1/2, Less Than2/2
  AND/1 -> brake/1
  Less Than2/1 -> AND/2
  <v_error>/1 -> Less Than2/1
  Less Than1/1 -> AND/1
  driver_input/1 -> Less Than1/1

== system car_model_5_28_2023/Driver & Environment/Reference Generator/Subsystem ==
  <psi> : Inport
  Constant1 : Constant  Value=2*pi
  Constant2 : Constant  Value=pi
  Constant3 : Constant  Value=-pi
  Constant4 : Constant  Value=2*pi
  Constant5 : Constant  Value=-2*pi
  GreaterThan : RelationalOperator  Operator=>  OutDataTypeStr=boolean  RndMeth=Simplest  InputSameDT=off
  Less Than : RelationalOperator  Operator=<  OutDataTypeStr=boolean  RndMeth=Simplest  InputSameDT=off
  Mod : Math  Operator=mod
  Product : Product
  Product1 : Product
  Sum : Sum  Inputs=+++
  psi_rev : Outport
  wires:
  Product1/1 -> Sum/3
  Less Than/1 -> Product1/2
  GreaterThan/1 -> Product/1
  Mod/1 -> GreaterThan/1, Sum/1, Less Than/1
  Constant1/1 -> Mod/2
  Constant5/1 -> Product/2
  Constant3/1 -> Less Than/2
  Constant4/1 -> Product1/1
  Constant2/1 -> GreaterThan/2
  Product/1 -> Sum/2
  Sum/1 -> psi_rev/1
  <psi>/1 -> Mod/1

== system car_model_5_28_2023/Vehicle Model/Electronics/Cooling Sensors ==
  Analog Signals : Inport
  Bus Creator9 : BusCreator  Inputs=5
  Bus Selector : BusSelector  OutputSignals=trn.motor_temperature,trn.mc_temp,trn.motor_fluid_temperature,trn.battery_temperature,trn.battery_fluid_temperature
  Delay1 : Delay  InitialCondition=[1 1; 1 1; 1 1; 1 1].*sim.IC.motor_T_IC
  Delay11 : Delay  InitialCondition=[1 1; 1 1; 1 1; 1 1].*sim.IC.motor_T_IC
  Delay12 : Delay  InitialCondition=[1 1; 1 1].*sim.IC.motor_FT_IC
  Delay13 : Delay  InitialCondition=[1 1].*sim.IC.battery_T_IC
  Delay14 : Delay  InitialCondition=[1 1].*sim.IC.battery_FT_IC
  Rate Transition1 : RateTransition  InitialCondition=[1 1].*sim.IC.motor_FT_IC  OutPortSampleTime=0
  Rate Transition2 : RateTransition  InitialCondition=sim.IC.battery_T_IC  OutPortSampleTime=0
  Rate Transition3 : RateTransition  InitialCondition=sim.IC.battery_FT_IC  OutPortSampleTime=0
  Saturation10 : Saturate  UpperLimit=sim.range.MOTOR_TEMPERATURE_MAX  LowerLimit=sim.range.MOTOR_TEMPERATURE_MIN
  Saturation11 : Saturate  UpperLimit=sim.range.BATTERY_TEMPERATURE_MAX  LowerLimit=sim.range.BATTERY_TEMPERATURE_MIN
  Saturation12 : Saturate  UpperLimit=sim.range.BATTERY_TEMPERATURE_MAX  LowerLimit=sim.range.BATTERY_TEMPERATURE_MIN
  Saturation18 : Saturate  UpperLimit=sim.range.MOTOR_TEMPERATURE_MAX  LowerLimit=sim.range.MOTOR_TEMPERATURE_MIN
  Saturation21 : Saturate  UpperLimit=sim.range.MOTOR_TEMPERATURE_MAX  LowerLimit=sim.range.MOTOR_TEMPERATURE_MIN
  Zero-Order Hold{1,11..14} (5 alike) : ZeroOrderHold  SampleTime=sim.timing.duplicate
  Cooling Sensors : Outport
  wires:
  Delay1/1 -> Saturation21/1
  Saturation21/1 -> Bus Creator9/2  "mc_T"
  Bus Selector/2 -> Zero-Order Hold1/1  "<mc_temp>"
  Zero-Order Hold1/1 -> Delay1/1
  Delay14/1 -> Saturation12/1
  Delay11/1 -> Saturation18/1
  Delay12/1 -> Saturation10/1
  Saturation12/1 -> Bus Creator9/5  "batt_FT"
  Zero-Order Hold12/1 -> Delay12/1
  Zero-Order Hold14/1 -> Delay14/1
  Bus Selector/4 -> Rate Transition2/1  "<battery_temperature>"
  Zero-Order Hold11/1 -> Delay11/1
  Saturation18/1 -> Bus Creator9/1  "motor_T"
  Zero-Order Hold13/1 -> Delay13/1
  Bus Selector/3 -> Rate Transition1/1  "<motor_fluid_temperature>"
  Saturation11/1 -> Bus Creator9/4  "batt_T"
  Saturation10/1 -> Bus Creator9/3  "motor_FT"
  Delay13/1 -> Saturation11/1
  Bus Selector/1 -> Zero-Order Hold11/1  "<motor_temperature>"
  Bus Selector/5 -> Rate Transition3/1  "<battery_fluid_temperature>"
  Bus Creator9/1 -> Cooling Sensors/1
  Rate Transition1/1 -> Zero-Order Hold12/1  "motor_fluid_temperature"
  Rate Transition2/1 -> Zero-Order Hold13/1  "battery_temperature"
  Rate Transition3/1 -> Zero-Order Hold14/1  "battery_fluid_temperature"
  Analog Signals/1 -> Bus Selector/1

== system car_model_5_28_2023/Vehicle Model/Electronics/Corner Dynamics Sensors ==
  Analog Signals : Inport
  Bus Creator10 : BusCreator  Inputs=4
  Bus Selector : BusSelector  OutputSignals=whl.TireFrame.Omega,sus.Sus.steering_angle,sus.Sus.shock_length,whl.TireFrame.GndFz
  Delay15 : Delay  InitialCondition=ones(1, 4, 2).*sim.IC.omega_IC
  Delay16 : Delay  InitialCondition=[1 1].*sim.IC.theta_IC
  Delay17 : Delay  InitialCondition=[1 1; 1 1; 1 1; 1 1].*sim.IC.shock_length_IC
  Delay18 : Delay  InitialCondition=[1 1; 1 1; 1 1; 1 1].*sim.IC.Fz_IC
  Saturation15 : Saturate  UpperLimit=sim.range.SHOCK_LENGTH_MAX  LowerLimit=sim.range.SHOCK_LENGTH_MIN
  Saturation16 : Saturate  UpperLimit=sim.range.OMEGA_MAX  LowerLimit=sim.range.OMEGA_MIN
  Saturation17 : Saturate  UpperLimit=sim.range.FZ_MAX  LowerLimit=sim.range.FZ_MIN
  Saturation3 : Saturate  UpperLimit=sim.range.CENTER_STEER_ANGLE_MAX  LowerLimit=-sim.range.CENTER_STEER_ANGLE_MAX
  Transpose : Math  Operator=transpose
  Zero-Order Hold{15..18} (4 alike) : ZeroOrderHold  SampleTime=sim.timing.duplicate
  Corner Dynamics Sensors : Outport
  wires:
  Transpose/1 -> Zero-Order Hold15/1  "omega"
  Bus Selector/1 -> Transpose/1  "<Omega>"
  Zero-Order Hold18/1 -> Delay18/1
  Delay18/1 -> Saturation17/1
  Zero-Order Hold15/1 -> Delay15/1
  Zero-Order Hold16/1 -> Delay16/1
  Saturation17/1 -> Bus Creator10/4  "FZ"
  Saturation3/1 -> Bus Creator10/2  "theta"
  Bus Selector/3 -> Zero-Order Hold17/1  "<shock_length>"
  Saturation15/1 -> Bus Creator10/3  "shock_L"
  Saturation16/1 -> Bus Creator10/1  "omega"
  Bus Selector/4 -> Zero-Order Hold18/1  "<GndFz>"
  Delay16/1 -> Saturation3/1
  Bus Selector/2 -> Zero-Order Hold16/1  "<steering_angle>"
  Delay17/1 -> Saturation15/1
  Delay15/1 -> Saturation16/1
  Zero-Order Hold17/1 -> Delay17/1
  Bus Creator10/1 -> Corner Dynamics Sensors/1
  Analog Signals/1 -> Bus Selector/1

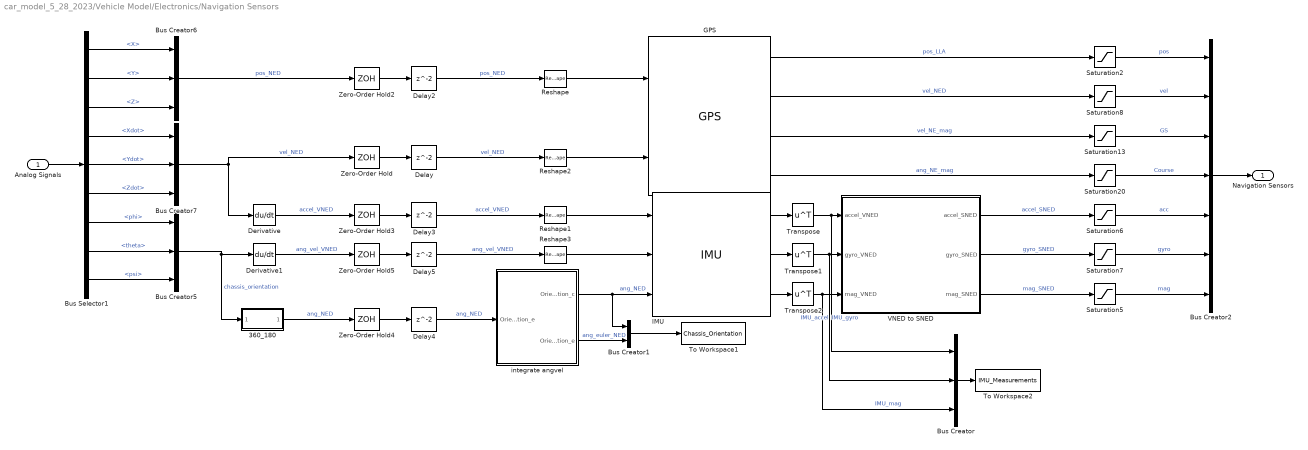
== system car_model_5_28_2023/Vehicle Model/Electronics/Navigation Sensors ==
  Analog Signals : Inport
  360_180 : Subsystem
  Bus Creator : BusCreator  Inputs=IMU_accel,IMU_gyro,IMU_mag
  Bus Creator1 : BusCreator  Inputs=2
  Bus Creator2 : BusCreator  Inputs=7
  Bus Creator5 : BusCreator  Inputs=phi,theta,psi
  Bus Creator6 : BusCreator  Inputs=X,Y,Z
  Bus Creator7 : BusCreator  Inputs=Xdot,Ydot,Zdot
  Bus Selector1 : BusSelector  OutputSignals=veh.InertFrm.Cg.Disp.X,veh.InertFrm.Cg.Disp.Y,veh.InertFrm.Cg.Disp.Z,veh.InertFrm.Cg.Vel.Xdot,veh.InertFrm.Cg.Vel.Ydot,veh.InertFrm.Cg.Vel.Zdot,veh.InertFrm.Cg.Ang.phi,veh.InertFrm.Cg.Ang.theta,veh.InertFrm.Cg.Ang.psi
  Delay : Delay  InitialCondition=([1;1]*sim.IC.vel_IC)'
  Delay2 : Delay  InitialCondition=[1 1; 1 1; 1 1].*sim.IC.pos_IC
  Delay3 : Delay  InitialCondition=[1 1; 1 1; 1 1].*sim.IC.acc_IC
  Delay4 : Delay  InitialCondition=[1 1; 1 1; 1 1].*sim.IC.ang_IC
  Delay5 : Delay  InitialCondition=[1 1; 1 1; 1 1].*sim.IC.ang_vel_IC
  Derivative : Derivative
  Derivative1 : Derivative
  GPS : sensorgpslib/GPS  DispRefFrame=NED  PositionInputFormat=Local  ReferenceLocation=sim.IC.location_lla_IC  HorizontalPositionAccuracy=sensor.gps.GPS_Z_ACCURACY  VerticalPositionAccuracy=sensor.gps.GPS_XY_ACCURACY  VelocityAccuracy=sensor.gps.GPS_V_ACCURACY  DecayFactor=sensor.gps.GPS_NOISE_FACTOR  SeedDouble=sensor.gps.r_GPS  SimulateUsing=Interpreted execution
      settings: LibrarySourceBlock=mspsensorlib/GPS
  IMU : mspsensorlib/IMU  DispRefFrame=NED  Temperature=25  MagneticFieldNED=sim.IC.mag_field_IC  MagneticFieldENU=[ -2.4169, 27.5550, 16.0849 ]  SeedDouble=sensor.imu.r_IMU  SimulateUsing=Interpreted execution  AccelParamsMeasurementRange=sensor.imu.ACC_MAX  AccelParamsResolution=sensor.imu.ACC_RES  AccelParamsConstantBias=sensor.imu.ACC_BIAS  AccelParamsAxesMisalignment=sensor.imu.ACC_SKEW  AccelParamsNoiseDensity=sensor.imu.ACC_VEL_WALK  AccelParamsBiasInstability=sensor.imu.ACC_BIAS_INSTABILITY  AccelParamsRandomWalk=sensor.imu.ACC_WALK  AccelParamsTemperatureBias=sensor.imu.ACC_T_BIAS  AccelParamsTemperatureScaleFactor=sensor.imu.ACC_T_SCALE  GyroParamsMeasurementRange=sensor.imu.GYR_MAX  GyroParamsResolution=sensor.imu.GYR_RES  GyroParamsConstantBias=sensor.imu.GYR_BIAS  GyroParamsAxesMisalignment=sensor.imu.GYR_SKEW  GyroParamsAccelerationBias=sensor.imu.GYR_ACC_BIAS  GyroParamsNoiseDensity=sensor.imu.GYR_ANG_WALK  GyroParamsBiasInstability=sensor.imu.GYR_BIAS_INSTABILITY  GyroParamsRandomWalk=sensor.imu.GYR_WALK  GyroParamsTemperatureBias=sensor.imu.GYR_T_BIAS  GyroParamsTemperatureScaleFactor=sensor.imu.GYR_T_SCALE  MagParamsMeasurementRange=sensor.imu.MAG_MAX  MagParamsResolution=sensor.imu.MAG_RES  MagParamsConstantBias=sensor.imu.MAG_BIAS  MagParamsAxesMisalignment=sensor.imu.MAG_SKEW  MagParamsNoiseDensity=sensor.imu.MAG_WHITE  MagParamsBiasInstability=sensor.imu.MAG_BIAS_INSTABILITY  MagParamsRandomWalk=sensor.imu.MAG_WALK  MagParamsTemperatureBias=sensor.imu.MAG_T_BIAS  MagParamsTemperatureScaleFactor=sensor.imu.MAG_T_SCALE
  Reshape{,1..3} (4 alike) : Reshape  OutputDimensionality=Row vector (2-D)
  Saturation13 : Saturate  UpperLimit=sim.range.VELOCITY_MAX  LowerLimit=-sim.range.VELOCITY_MAX
  Saturation2 : Saturate  UpperLimit=inf  LowerLimit=-inf
  Saturation20 : Saturate  UpperLimit=sim.range.ORIENTATION_MAX  LowerLimit=-sim.range.ORIENTATION_MAX
  Saturation5 : Saturate  UpperLimit=sim.range.MAG_MAX  LowerLimit=-sim.range.MAG_MAX
  Saturation6 : Saturate  UpperLimit=sim.range.ACCELERATION_MAX  LowerLimit=-sim.range.ACCELERATION_MAX
  Saturation7 : Saturate  UpperLimit=sim.range.YAW_MAX  LowerLimit=-sim.range.YAW_MAX
  Saturation8 : Saturate  UpperLimit=sim.range.VELOCITY_MAX  LowerLimit=-sim.range.VELOCITY_MAX
  To Workspace1 : ToWorkspace  VariableName=Chassis_Orientation  SaveFormat=Timeseries  SampleTime=-1
  To Workspace2 : ToWorkspace  VariableName=IMU_Measurements  SaveFormat=Timeseries  SampleTime=-1
  Transpose : Math  Operator=transpose
  Transpose1 : Math  Operator=transpose
  Transpose2 : Math  Operator=transpose
  VNED to SNED : MATLAB Function  TreatAsAtomicUnit=on
  Zero-Order Hold{,2..5} (5 alike) : ZeroOrderHold  SampleTime=sim.timing.duplicate
  integrate angvel : MATLAB Function  TreatAsAtomicUnit=on
  Navigation Sensors : Outport
  wires:
  Delay5/1 -> Reshape3/1  "ang_vel_VNED"
  Delay/1 -> Reshape2/1  "vel_NED"
  Delay3/1 -> Reshape1/1  "accel_VNED"
  Delay2/1 -> Reshape/1  "pos_NED"
  integrate angvel/1(Orientation_c) -> Bus Creator1/1, IMU/3  "ang_NED"
  GPS/4 -> Saturation20/1  "ang_NE_mag"
  GPS/3 -> Saturation13/1  "vel_NE_mag"
  GPS/2 -> Saturation8/1  "vel_NED"
  GPS/1 -> Saturation2/1  "pos_LLA"
  VNED to SNED/2(gyro_SNED) -> Saturation7/1  "gyro_SNED"
  VNED to SNED/1(accel_SNED) -> Saturation6/1  "accel_SNED"
  VNED to SNED/3(mag_SNED) -> Saturation5/1  "mag_SNED"
  Delay4/1 -> integrate angvel/1("Orientation_e ")  "ang_NED"
  Transpose2/1 -> Bus Creator/3, VNED to SNED/3(mag_VNED)  "IMU_mag"
  Transpose1/1 -> Bus Creator/2, VNED to SNED/2(gyro_VNED)  "IMU_gyro"
  Transpose/1 -> Bus Creator/1, VNED to SNED/1(accel_VNED)  "IMU_accel"
  IMU/3 -> Transpose2/1
  IMU/1 -> Transpose/1
  IMU/2 -> Transpose1/1
  Bus Creator/1 -> To Workspace2/1
  Bus Creator1/1 -> To Workspace1/1
  integrate angvel/2(Orientation_e) -> Bus Creator1/2  "ang_euler_NED"
  Zero-Order Hold/1 -> Delay/1
  Bus Creator7/1 -> Zero-Order Hold/1, Derivative/1  "vel_NED"
  Zero-Order Hold2/1 -> Delay2/1
  Bus Creator6/1 -> Zero-Order Hold2/1  "pos_NED"
  Zero-Order Hold3/1 -> Delay3/1
  Derivative/1 -> Zero-Order Hold3/1  "accel_VNED"
  Zero-Order Hold5/1 -> Delay5/1
  Derivative1/1 -> Zero-Order Hold5/1  "ang_vel_VNED"
  Zero-Order Hold4/1 -> Delay4/1
  360_180/1(psi_rev) -> Zero-Order Hold4/1  "ang_NED"
  Saturation2/1 -> Bus Creator2/1  "pos"
  Saturation13/1 -> Bus Creator2/3  "GS"
  Saturation6/1 -> Bus Creator2/5  "acc"
  Saturation20/1 -> Bus Creator2/4  "Course"
  Saturation5/1 -> Bus Creator2/7  "mag"
  Saturation8/1 -> Bus Creator2/2  "vel"
  Saturation7/1 -> Bus Creator2/6  "gyro"
  Bus Creator2/1 -> Navigation Sensors/1
  Bus Selector1/1 -> Bus Creator6/1  "<X>"
  Bus Selector1/8 -> Bus Creator5/2  "<theta>"
  Bus Selector1/2 -> Bus Creator6/2  "<Y>"
  Bus Selector1/6 -> Bus Creator7/3  "<Zdot>"
  Bus Selector1/5 -> Bus Creator7/2  "<Ydot>"
  Bus Selector1/4 -> Bus Creator7/1  "<Xdot>"
  Bus Selector1/7 -> Bus Creator5/1  "<phi>"
  Bus Creator5/1 -> 360_180/1(<psi>), Derivative1/1  "chassis_orientation"
  Bus Selector1/3 -> Bus Creator6/3  "<Z>"
  Bus Selector1/9 -> Bus Creator5/3  "<psi>"
  Analog Signals/1 -> Bus Selector1/1
  Reshape/1 -> GPS/1
  Reshape1/1 -> IMU/1
  Reshape2/1 -> GPS/2
  Reshape3/1 -> IMU/2

== system car_model_5_28_2023/Vehicle Model/Electronics/Power Sensors ==
  Analog Signals : Inport
  Bus Creator8 : BusCreator  Inputs=5
  Bus Selector : BusSelector  OutputSignals=trn.battery_voltage,trn.battery_current,trn.motor_voltage,trn.motor_current,trn.power_limits
  Delay10 : Delay  InitialCondition=[sim.IC.dcl_IC; sim.IC.ccl_IC]*[1 1]
  Delay6 : Delay  InitialCondition=[1 1].*sim.IC.battery_voltage_IC
  Delay7 : Delay  InitialCondition=[1 1].*sim.IC.battery_current_IC
  Delay8 : Delay  InitialCondition=ones(1, 4, 2).*sim.IC.motor_voltage_IC
  Delay9 : Delay  InitialCondition=ones(1, 4, 2).*sim.IC.motor_current_IC
  Saturation1 : Saturate  UpperLimit=sim.range.BATTERY_CURRENT_MAX  LowerLimit=sim.range.BATTERY_CURRENT_MIN
  Saturation14 : Saturate  UpperLimit=sim.range.DCL_MAX  LowerLimit=sim.range.DCL_MIN
  Saturation19 : Saturate  UpperLimit=sim.range.BATTERY_VOLTAGE_MAX  LowerLimit=sim.range.BATTERY_VOLTAGE_MIN
  Saturation4 : Saturate  UpperLimit=sim.range.MOTOR_VOLTAGE_MAX  LowerLimit=sim.range.MOTOR_VOLTAGE_MIN
  Saturation9 : Saturate  UpperLimit=sim.range.MOTOR_CURRENT_MAX  LowerLimit=sim.range.MOTOR_CURRENT_MIN
  Zero-Order Hold{6..10} (5 alike) : ZeroOrderHold  SampleTime=sim.timing.duplicate
  Power Sensors : Outport
  wires:
  Zero-Order Hold6/1 -> Delay6/1
  Delay6/1 -> Saturation19/1
  Bus Selector/1 -> Zero-Order Hold6/1  "<battery_voltage>"
  Delay7/1 -> Saturation1/1
  Zero-Order Hold7/1 -> Delay7/1
  Bus Selector/2 -> Zero-Order Hold7/1  "<battery_current>"
  Delay8/1 -> Saturation4/1
  Zero-Order Hold8/1 -> Delay8/1
  Bus Selector/3 -> Zero-Order Hold8/1  "<motor_voltage>"
  Delay9/1 -> Saturation9/1
  Zero-Order Hold9/1 -> Delay9/1
  Bus Selector/4 -> Zero-Order Hold9/1  "<motor_current>"
  Zero-Order Hold10/1 -> Delay10/1
  Delay10/1 -> Saturation14/1
  Bus Selector/5 -> Zero-Order Hold10/1  "<power_limits>"
  Saturation19/1 -> Bus Creator8/1  "batt_V"
  Saturation1/1 -> Bus Creator8/2  "batt_I"
  Saturation9/1 -> Bus Creator8/4  "motor_I"
  Saturation4/1 -> Bus Creator8/3  "motor_V"
  Saturation14/1 -> Bus Creator8/5  "pwr_lmt"
  Bus Creator8/1 -> Power Sensors/1
  Analog Signals/1 -> Bus Selector/1

== system car_model_5_28_2023/Vehicle Model/Powertrain/Battery Cooling Loop ==
  omega_m : Inport
  Battery_V : Inport  Port=2
  Battery_I : Inport  Port=3
  CL Battery Fans : Inport  Port=4
  CL Battery Pump : Inport  Port=5
  Vg : Inport  Port=6
  Battery Temperature : Outport
  Battery Fluid Temperature : Outport  Port=2

== system car_model_5_28_2023/Vehicle Model/Powertrain/Drivetrain ==
  battery voltage : Inport
  throttle : Inport  Port=2
  motor speed : Inport  Port=3
  1-D Lookup Table : Lookup_n-D  NumberOfTableDimensions=1  LookupTableObject=''  BreakpointsForDimension1=powertrain.motor.speed_bp  BreakpointsForDimension1FirstPoint=10  BreakpointsForDimension2FirstPoint=10  BreakpointsForDimension1Spacing=12  BreakpointsForDimension2Spacing=12  BeginIndexSearchUsingPreviousIndexResult=on  Table=powertrain.motor.max_torque_table  ExtrapMethod=Clip  DiagnosticForOutOfRangeInput=Error  InternalRulePriority=Speed  RndMeth=Simplest
  1-D Lookup Table1 : Lookup_n-D  NumberOfTableDimensions=1  LookupTableObject=''  BreakpointsForDimension1=powertrain.motor.speed_bp  BreakpointsForDimension1FirstPoint=10  BreakpointsForDimension2FirstPoint=10  BreakpointsForDimension1Spacing=12  BreakpointsForDimension2Spacing=12  BeginIndexSearchUsingPreviousIndexResult=on  Table=powertrain.motor.max_current_table  ExtrapMethod=Clip  DiagnosticForOutOfRangeInput=Error  InternalRulePriority=Speed  RndMeth=Simplest
  Gain : Gain  Gain=sim.top_parameters.MOTOR_ENABLE
  Gain1 : Gain  Gain=powertrain.gearbox.gr.*powertrain.gearbox.ge
  Gain2 : Gain  Gain=sim.top_parameters.MOTOR_ENABLE
  Mean : dspstat3/Mean  run=off  InputProcessing=Columns as channels (frame based)  reset_popup=None  directionMode=Entire input  dimension=1  roiEnable=off  roiType=Rectangles  roiPortion=Entire ROI  roiOutput=Individual statistics for each ROI  roiFlag=off  roundingMode=Floor  overflowMode=off  outputDataTypeStr=Inherit: Same as accumulator  outputMin=[]  outputMax=[]  outputLastDataTypeStr=Inherit: Same as accumulator
  Product : Product
  Product1 : Product
  Sum : Sum  Inputs=+
  Terminator : Terminator
  battery current : Outport
  motor current : Outport  Port=2
  wheel torque : Outport  Port=3
  motor torque : Outport  Port=4
  wires:
  1-D Lookup Table/1 -> Gain/1
  motor speed/1 -> 1-D Lookup Table1/1, Mean/1
  Product/1 -> motor torque/1, Gain1/1
  throttle/1 -> Product/1, Product1/1
  Gain/1 -> Product/2
  Gain1/1 -> wheel torque/1
  Sum/1 -> battery current/1
  battery voltage/1 -> Terminator/1
  Mean/1 -> 1-D Lookup Table/1
  1-D Lookup Table1/1 -> Gain2/1
  Gain2/1 -> Product1/2
  Product1/1 -> motor current/1, Sum/1

== system car_model_5_28_2023/Vehicle Model/Powertrain/HV Battery ==
  battery_I : Inport
  1-D Lookup Table : Lookup_n-D  NumberOfTableDimensions=1  BreakpointsForDimension1=powertrain.battery.SOC  Table=powertrain.battery.Em  InternalRulePriority=Speed  RndMeth=Simplest
  Constant1 : Constant  Value=sim.IC.SOC_IC
  Gain : Gain  Gain=1/(3600*powertrain.battery.Np*powertrain.battery.Ah)
  Gain1 : Gain  Gain=powertrain.battery.Ns
  Gain2 : Gain  Gain=powertrain.battery.R
  Integrator : Integrator
  Sum1 : Sum  Inputs=|+-
  Sum2 : Sum  Inputs=|+-
  battery_V : Outport
  wires:
  Gain/1 -> Sum1/2
  Constant1/1 -> Sum1/1
  Gain2/1 -> Sum2/2
  Integrator/1 -> Gain/1
  Sum2/1 -> battery_V/1
  battery_I/1 -> Gain2/1, Integrator/1
  Sum1/1 -> 1-D Lookup Table/1  "SOC"
  1-D Lookup Table/1 -> Gain1/1
  Gain1/1 -> Sum2/1
